simulink model "simplePendulumSample"  (R2017b)
settings: Solver=VariableStepAuto  StartTime=0.0  StopTime=10.0  RelTol=1e-3
values from neighbouring files (symbols this model uses):
  g = 9.82    [forceTest.m]    (also in initPendulum.m; plotCartPendulumAnimationOde45.m; simSimpleOdeFun.m; simpleOdeFunSample.m)
  l = 0.3348    [initPendulum.m]    (also in plotCartPendulumAnimationOde45.m = 0.647; pplane8.m = l+1; simSimpleOdeFun.m = 1; simpleOdeFunSample.m = 1)
  m = 4+.100+.075+.026    (= 4.201)    [initPendulum.m]    (also in plotCartPendulumAnimationOde45.m = 0.402; simSimpleOdeFun.m = 1; simpleOdeFunSample.m = 1; testScr.m = 1)
settings Model: Creator=niels  LastModifiedBy=niels
settings DataIOCC: Refine=3

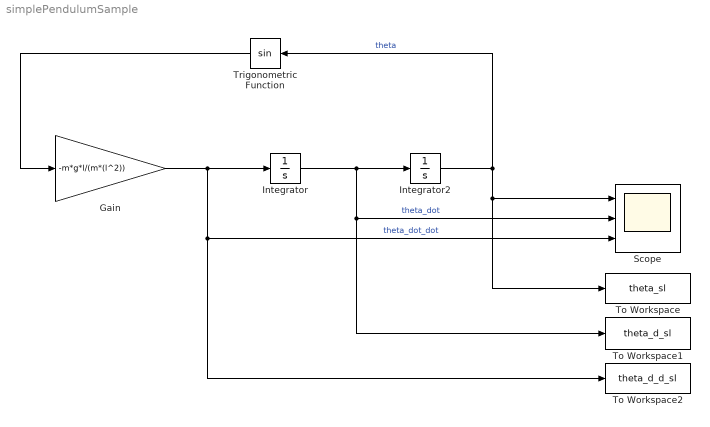
== system simplePendulumSample ==
  Gain : Gain  Gain=-m*g*l/(m*(l^2))
  Integrator : Integrator
  Integrator2 : Integrator  InitialCondition=pi/2
  Scope : Scope  NumInputPorts=3
  To Workspace : ToWorkspace  VariableName=theta_sl  SaveFormat=Timeseries  SampleTime=-1
  To Workspace1 : ToWorkspace  VariableName=theta_d_sl  SaveFormat=Timeseries  SampleTime=-1
  To Workspace2 : ToWorkspace  VariableName=theta_d_d_sl  SaveFormat=Timeseries  SampleTime=-1
  Trigonometric Function : Trigonometry
  wires:
  Integrator/1 -> Scope/2, To Workspace1/1, Integrator2/1  "theta_dot"
  Integrator2/1 -> Trigonometric Function/1, Scope/1, To Workspace/1  "theta"
  Gain/1 -> To Workspace2/1, Scope/3, Integrator/1  "theta_dot_dot"
  Trigonometric Function/1 -> Gain/1
